simulink model "cvoo_g19_lqr_por_cima_do_sae"  (R2020a)
settings: Solver=VariableStepAuto  StartTime=0.0  StopTime=10.0  RelTol=1e-3
values from neighbouring files (symbols this model uses):
  a_h = [ ... (first row only)    [main.m]    (also in main_gaspar.m)
  b_h_sf = b_h(:,[1,3])    [main.m]    (also in main_gaspar.m)
  c_h = eye(size(a_h))    [main.m]    (also in main_gaspar.m)
  d_h_sf = d_h(:,[1,3])    [main.m]    (also in main_gaspar.m)
  h_ref = fscanf(fileID,'    [ground_model.m]
  K_lqr = lqr(a_h_pt_int, b_h_pt_int, Q, R)    [main.m]    (also in main_gaspar.m = lqr(a_h_int, b_h_sf_int, Q, R))
  k_u_dsp = 0.65    [main.m]    (also in main_gaspar.m)
  k_w_dsp = 4.1    [main.m]    (also in main_gaspar.m)
  x0 = [0 0 0 0]    [main.m]    (also in main_gaspar.m)
undefined symbols (not defined in the file or in its folder): max_deflec
settings Model: Creator=josem  LastModifiedBy=josem

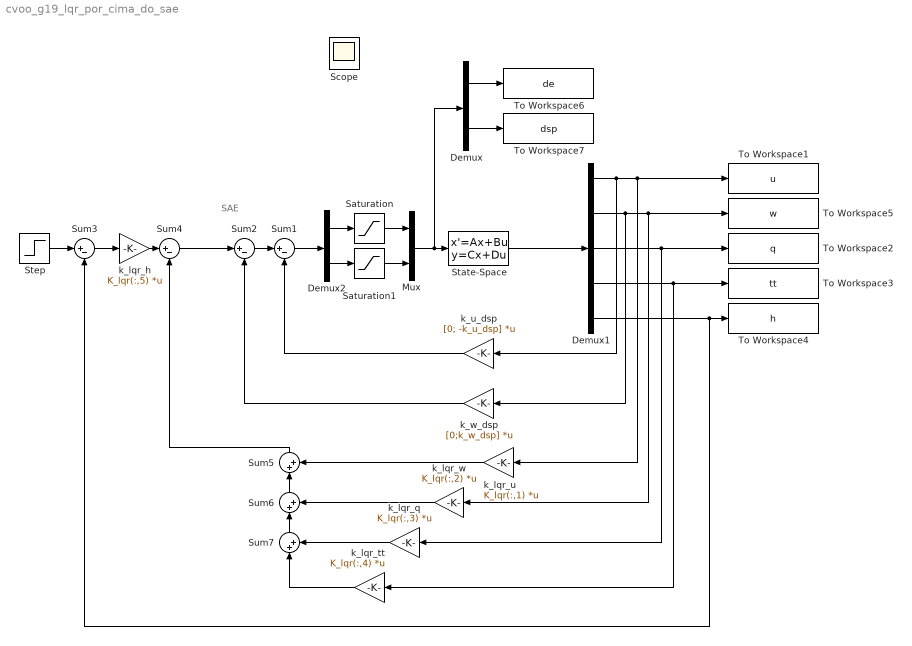
== system cvoo_g19_lqr_por_cima_do_sae ==
  note: SAE
  Demux : Demux  Outputs=2
  Demux1 : Demux  Outputs=5
  Demux2 : Demux  Outputs=2
  Mux : Mux  Inputs=2
  Saturation : Saturate  UpperLimit=max_deflec.demax  LowerLimit=max_deflec.demin
  Saturation1 : Saturate  UpperLimit=max_deflec.spmax  LowerLimit=0
  State-Space : StateSpace  A=a_h  B=b_h_sf  C=c_h  D=d_h_sf  InitialCondition=x0
  Step : Step  After=h_ref  SampleTime=0  VectorParams1D=off
  Sum{1..4} (4 alike) : Sum  Inputs=|+-
  Sum5 : Sum  Inputs=|++
  Sum6 : Sum  Inputs=|++
  Sum7 : Sum  Inputs=|++
  To Workspace1 : ToWorkspace  VariableName=u  SampleTime=-1
  To Workspace2 : ToWorkspace  VariableName=q  SampleTime=-1
  To Workspace3 : ToWorkspace  VariableName=tt  SampleTime=-1
  To Workspace4 : ToWorkspace  VariableName=h  SampleTime=-1
  To Workspace5 : ToWorkspace  VariableName=w  SampleTime=-1
  To Workspace6 : ToWorkspace  VariableName=de  SampleTime=-1
  To Workspace7 : ToWorkspace  VariableName=dsp  SampleTime=-1
  k_lqr_h : Gain  Gain=K_lqr(:,5)  Multiplication=Matrix(K*u)
  k_lqr_q : Gain  Gain=K_lqr(:,3)  Multiplication=Matrix(K*u)
  k_lqr_tt : Gain  Gain=K_lqr(:,4)  Multiplication=Matrix(K*u)
  k_lqr_u : Gain  Gain=K_lqr(:,1)  Multiplication=Matrix(K*u)
  k_lqr_w : Gain  Gain=K_lqr(:,2)  Multiplication=Matrix(K*u)
  k_u_dsp : Gain  Gain=[0; -k_u_dsp]  Multiplication=Matrix(K*u)
  k_w_dsp : Gain  Gain=[0;k_w_dsp]  Multiplication=Matrix(K*u)
  Scope : Scope
  wires:
  State-Space/1 -> Demux1/1
  Demux1/2 -> k_w_dsp/1, k_lqr_w/1, To Workspace5/1
  Demux1/1 -> k_u_dsp/1, k_lqr_u/1, To Workspace1/1
  Demux1/3 -> k_lqr_q/1, To Workspace2/1
  Demux1/4 -> k_lqr_tt/1, To Workspace3/1
  Demux1/5 -> Sum3/2, To Workspace4/1
  k_u_dsp/1 -> Sum1/2
  Sum2/1 -> Sum1/1
  k_w_dsp/1 -> Sum2/2
  Step/1 -> Sum3/1
  Sum3/1 -> k_lqr_h/1
  k_lqr_h/1 -> Sum4/1
  Sum6/1 -> Sum5/1
  k_lqr_w/1 -> Sum6/2
  Sum7/1 -> Sum6/1
  k_lqr_q/1 -> Sum7/2
  k_lqr_tt/1 -> Sum7/1
  Sum5/1 -> Sum4/2
  Demux/1 -> To Workspace6/1
  Demux/2 -> To Workspace7/1
  k_lqr_u/1 -> Sum5/2
  Saturation1/1 -> Mux/2
  Demux2/2 -> Saturation1/1
  Demux2/1 -> Saturation/1
  Saturation/1 -> Mux/1
  Sum4/1 -> Sum2/1
  Sum1/1 -> Demux2/1
  Mux/1 -> Demux/1, State-Space/1
